simulink model "Six_phase_inverter"  (R2014b)
settings: Solver=ode23tb  StartTime=0.0  StopTime=0.05  MaxStep=1e-4  RelTol=1e-3
InitFcn:
  | Vm=100;
  | Fc=3000;
libraries: powerlib x12, simulink_extras x1, simulink x1
settings Model: Creator=y  LastModifiedBy=Lei
settings DataIOCC: SignalLoggingSaveFormat=ModelDataLogs
settings OptimizationCC: ExpressionDepthLimit=2147483647  InitFltsAndDblsToZero=on
settings DebuggingCC: SaveWithParameterizedLinksMsg=none  UnderspecifiedInitializationDetection=Classic  MergeDetectMultiDrivingBlocksExec=none  SignalResolutionControl=TryResolveAllWithWarning  MultiTaskDSMMsg=warning  MultiTaskCondExecSysMsg=none  FcnCallInpInsideContextMsg=UseLocalSettings  StateNameClashWarn=warning
settings RTWCC: IncludeERTFirstTime=on
settings GRTTargetCC: TargetFcnLib=ansi_tfl_tmw.mat  CombineOutputUpdateFcns=off  GRTInterface=on

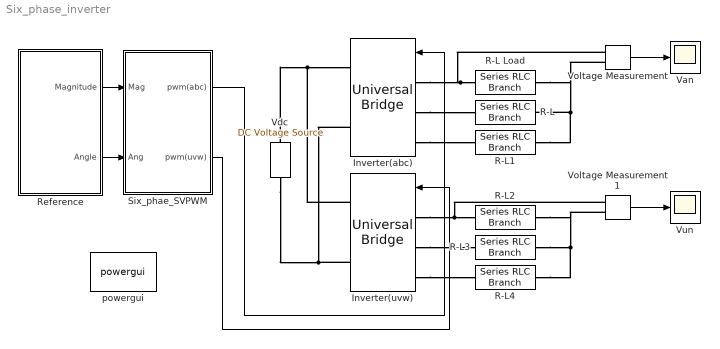
== system Six_phase_inverter ==
  Inverter(abc) : powerlib/Power Electronics/Universal Bridge  Arms=3  SnubberResistance=1e5  SnubberCapacitance=inf  Device=IGBT / Diodes  Ron=1e-3  Lon=0  ForwardVoltages="[  0  0  ]"  ForwardVoltage=0  GTOparameters=[ 10e-6 , 20e-6 ]  IGBTparameters=[ 1e-6 , 2e-6 ]  Measurements=None  Measurements_2=None  converterType=Rectifier
  Inverter(uvw) : powerlib/Power Electronics/Universal Bridge  Arms=3  SnubberResistance=1e5  SnubberCapacitance=inf  Device=IGBT / Diodes  Ron=1e-3  Lon=0  ForwardVoltages="[  0  0  ]"  ForwardVoltage=0  GTOparameters=[ 10e-6 , 20e-6 ]  IGBTparameters=[ 1e-6 , 2e-6 ]  Measurements=None  Measurements_2=None  converterType=Rectifier
  R-L{,1..4} (5 alike) : powerlib/Elements/Series RLC Branch  LConnTagsString=__new0  RConnTagsString=__new0  BranchType=RL  Resistance=10  Inductance=1e-03  SetiL0=off  InitialCurrent=0  Capacitance=[]  Setx0=off  InitialVoltage=0  Measurements=None
  R-L Load : powerlib/Elements/Series RLC Branch  LConnTagsString=__new0  RConnTagsString=__new0  BranchType=RL  Resistance=10  Inductance=1e-03  SetiL0=off  InitialCurrent=0  Capacitance=[]  Setx0=off  InitialVoltage=0  Measurements=None
  Reference : Subsystem
      mask Display:
      | disp('reference\nvoltage\ngenerator')
      | port_label('output',1,'mag')
      | port_label('output',2,'angle')
  Six_phae_SVPWM : Subsystem
  Van : Scope
      settings: TimeRange=0.05  YMin=-200  YMax=200  SaveName=Van  SampleInput=on  SampleTime=1e-6
  Vdc : powerlib/Electrical Sources/DC Voltage Source  Amplitude=300  Measurements=None
  Voltage Measurement : powerlib/Measurements/Voltage Measurement  PhasorSimulation=off  OutputType=Complex  PSBequivalent=0
  Voltage Measurement1 : powerlib/Measurements/Voltage Measurement  PhasorSimulation=off  OutputType=Complex  PSBequivalent=0
  Vun : Scope
      settings: YMin=-200  YMax=200  SaveName=Vbn  SampleInput=on  SampleTime=1e-6
  powergui : powerlib/powergui  Priority=1  SimulationMode=Continuous  SolverType=Tustin/Backward Euler (TBE)  SampleTime=50e-6  frequency=60  SPID=off  DisableSnubberDevices=off  DisableRonSwitches=off  DisableVfSwitches=off  SwTol=0  DisplayEquations=off  Interpol=off  methode=off  Ts=100  frequencyindice=0  Pbase=100e6  ErrMax=1e-4  Iterations=50  UnitsV=kV  UnitsW=MW  FunctionMessages=off  echomessages=off  HookPort=off  EnableUseOfTLC=off  x0status=blocks  RestoreLinks=warning  ResistiveCurrentMeasurement=off  Frange=[0:2:500]  Ylog=off  Xlog=on  ShowGrid=off  save=off  variable=ZData  structure=0  ZoomFFT=off  StartTime=0.0  cycles=1  DisplayStyle=1  fundamental=60  FreqAxis=off  MaxFrequency=1000  frequencyindicesteady=1  RmsSteady=1  display=off
  wires:
  Voltage Measurement/1 -> Van/1
  Reference/2(Angle) -> Six_phae_SVPWM/2(Ang)
  Reference/1(Magnitude) -> Six_phae_SVPWM/1(Mag)
  Voltage Measurement1/1 -> Vun/1
  Six_phae_SVPWM/1(pwm(abc)) -> Inverter(abc)/1
  Six_phae_SVPWM/2(pwm(uvw)) -> Inverter(uvw)/1
  connections:
  R-L Load/LConn1 -- Inverter(abc)/LConn1 -- Voltage Measurement/LConn1
  Inverter(abc)/LConn2 -- R-L/LConn1
  Inverter(abc)/LConn3 -- R-L1/LConn1
  Voltage Measurement1/LConn1 -- Inverter(uvw)/LConn1 -- R-L2/LConn1
  Inverter(uvw)/LConn2 -- R-L3/LConn1
  Inverter(uvw)/LConn3 -- R-L4/LConn1
  R-L4/RConn1 -- Voltage Measurement1/LConn2 -- R-L2/RConn1 -- R-L3/RConn1
  R-L1/RConn1 -- Voltage Measurement/LConn2 -- R-L Load/RConn1 -- R-L/RConn1
  Vdc/RConn1 -- Inverter(uvw)/RConn1 -- Inverter(abc)/RConn1
  Vdc/LConn1 -- Inverter(uvw)/RConn2 -- Inverter(abc)/RConn2

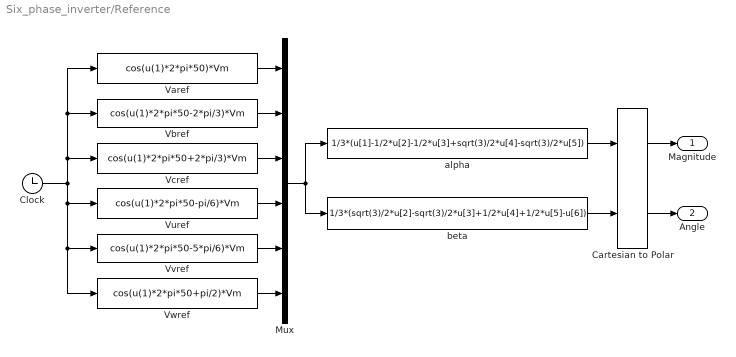
== system Six_phase_inverter/Reference ==
  Cartesian to Polar : simulink_extras/Transformations/Cartesian to Polar
  Clock : Clock
  Mux : Mux  Inputs=6
  Varef : Fcn  Expr=cos(u(1)*2*pi*50)*Vm
  Vbref : Fcn  Expr=cos(u(1)*2*pi*50-2*pi/3)*Vm
  Vcref : Fcn  Expr=cos(u(1)*2*pi*50+2*pi/3)*Vm
  Vuref : Fcn  Expr=cos(u(1)*2*pi*50-pi/6)*Vm
  Vvref : Fcn  Expr=cos(u(1)*2*pi*50-5*pi/6)*Vm
  Vwref : Fcn  Expr=cos(u(1)*2*pi*50+pi/2)*Vm
  alpha : Fcn  Expr=1/3*(u[1]-1/2*u[2]-1/2*u[3]+sqrt(3)/2*u[4]-sqrt(3)/2*u[5])
  beta : Fcn  Expr=1/3*(sqrt(3)/2*u[2]-sqrt(3)/2*u[3]+1/2*u[4]+1/2*u[5]-u[6])
  Magnitude : Outport
  Angle : Outport  Port=2
  wires:
  Varef/1 -> Mux/1
  Cartesian to Polar/1 -> Magnitude/1
  Cartesian to Polar/2 -> Angle/1
  Clock/1 -> Varef/1, Vbref/1, Vcref/1, Vwref/1, Vvref/1, Vuref/1
  Vbref/1 -> Mux/2
  Vcref/1 -> Mux/3
  Vvref/1 -> Mux/5
  Vwref/1 -> Mux/6
  Vuref/1 -> Mux/4
  Mux/1 -> alpha/1, beta/1
  beta/1 -> Cartesian to Polar/2
  alpha/1 -> Cartesian to Polar/1

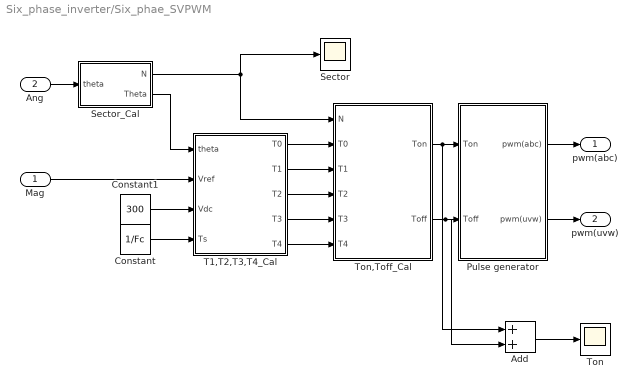
== system Six_phase_inverter/Six_phae_SVPWM ==
  Mag : Inport
  Ang : Inport  Port=2
  Add : Sum
  Constant : Constant  Value=1/Fc
  Constant1 : Constant  Value=300
  Pulse generator : Subsystem
  Sector : Scope
      settings: YMin=0  YMax=12  SaveName=N  SampleInput=on  SampleTime=1e-6
  Sector_Cal : Subsystem
  T1,T2,T3,T4_Cal : MATLAB Function  TreatAsAtomicUnit=on
  Ton : Scope
      settings: YMin=0  YMax=12  SaveName=Ton  SampleInput=on  SampleTime=1e-6
  Ton,Toff_Cal : MATLAB Function  TreatAsAtomicUnit=on
  pwm(abc) : Outport
  pwm(uvw) : Outport  Port=2
  wires:
  Sector_Cal/1(N) -> Ton,Toff_Cal/1(N), Sector/1
  Sector_Cal/2(Theta) -> T1,T2,T3,T4_Cal/1(theta)
  Constant1/1 -> T1,T2,T3,T4_Cal/3(Vdc)
  Constant/1 -> T1,T2,T3,T4_Cal/4(Ts)
  T1,T2,T3,T4_Cal/1(T0) -> Ton,Toff_Cal/2(T0)
  T1,T2,T3,T4_Cal/2(T1) -> Ton,Toff_Cal/3(T1)
  T1,T2,T3,T4_Cal/3(T2) -> Ton,Toff_Cal/4(T2)
  T1,T2,T3,T4_Cal/4(T3) -> Ton,Toff_Cal/5(T3)
  T1,T2,T3,T4_Cal/5(T4) -> Ton,Toff_Cal/6(T4)
  Ton,Toff_Cal/1(Ton) -> Add/1, Pulse generator/1(Ton)
  Ton,Toff_Cal/2(Toff) -> Add/2, Pulse generator/2(Toff)
  Ang/1 -> Sector_Cal/1(theta)
  Mag/1 -> T1,T2,T3,T4_Cal/2(Vref)
  Pulse generator/2(pwm(uvw)) -> pwm(uvw)/1
  Pulse generator/1(pwm(abc)) -> pwm(abc)/1
  Add/1 -> Ton/1

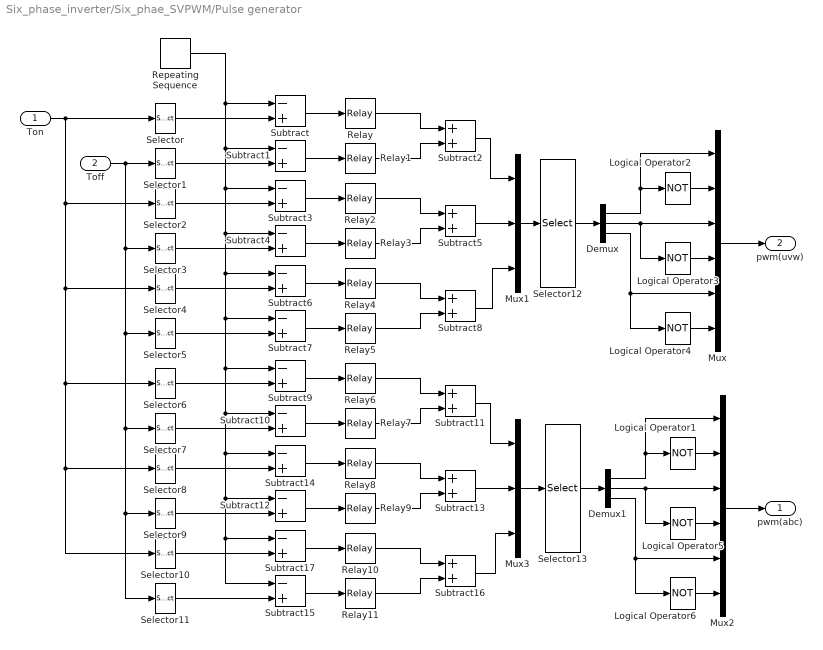
== system Six_phase_inverter/Six_phae_SVPWM/Pulse generator ==
  Ton : Inport
  Toff : Inport  Port=2
  Demux : Demux  Outputs=3
  Demux1 : Demux  Outputs=3
  Logical Operator{1..6} (6 alike) : Logic  Operator=NOT  OutDataTypeStr=float('double')
  Mux : Mux  Inputs=6
  Mux1 : Mux  Inputs=3
  Mux2 : Mux  Inputs=6
  Mux3 : Mux  Inputs=3
  Relay : Relay  OffSwitchValue=-eps
  Relay{1,3,5,7,9,11} (6 alike) : Relay  OnOutputValue=0  OffOutputValue=-1
  Relay{2,4,6,8,10} (5 alike) : Relay
  Repeating Sequence : simulink/Sources/Repeating Sequence  rep_seq_t=[0 0.5/Fc 1/Fc]  rep_seq_y=[0 0.5/Fc 0]
  Selector : Selector  InputPortWidth=6  Indices=[1]
  Selector1 : Selector  InputPortWidth=6  Indices=[1]
  Selector10 : Selector  InputPortWidth=6  Indices=[6]
  Selector11 : Selector  InputPortWidth=6  Indices=[6]
  Selector12 : Selector  InputPortWidth=3  Indices=[3 2 1]
  Selector13 : Selector  InputPortWidth=3  Indices=[3 2 1]
  Selector2 : Selector  InputPortWidth=6  Indices=[2]
  Selector3 : Selector  InputPortWidth=6  Indices=[2]
  Selector4 : Selector  InputPortWidth=6  Indices=[3]
  Selector5 : Selector  InputPortWidth=6  Indices=[3]
  Selector6 : Selector  InputPortWidth=6  Indices=[4]
  Selector7 : Selector  InputPortWidth=6  Indices=[4]
  Selector8 : Selector  InputPortWidth=6  Indices=[5]
  Selector9 : Selector  InputPortWidth=6  Indices=[5]
  Subtract{,1,3..4,6..7,9..10,12,14..15,17} (12 alike) : Sum  Inputs=-+
  Subtract{2,5,8,11,13,16} (6 alike) : Sum
  pwm(abc) : Outport
  pwm(uvw) : Outport  Port=2
  wires:
  Ton/1 -> Selector/1, Selector2/1, Selector4/1, Selector6/1, Selector8/1, Selector10/1
  Repeating Sequence/1 -> Subtract/1, Subtract1/1, Subtract3/1, Subtract4/1, Subtract6/1, Subtract7/1, Subtract9/1, Subtract10/1, Subtract14/1, Subtract12/1, Subtract15/1, Subtract17/1
  Subtract/1 -> Relay/1
  Toff/1 -> Selector9/1, Selector11/1, Selector7/1, Selector5/1, Selector3/1, Selector1/1
  Subtract1/1 -> Relay1/1
  Selector/1 -> Subtract/2
  Selector1/1 -> Subtract1/2
  Relay/1 -> Subtract2/1
  Relay1/1 -> Subtract2/2
  Subtract2/1 -> Mux1/1
  Subtract3/1 -> Relay2/1
  Subtract4/1 -> Relay3/1
  Selector2/1 -> Subtract3/2
  Selector3/1 -> Subtract4/2
  Relay2/1 -> Subtract5/1
  Relay3/1 -> Subtract5/2
  Subtract5/1 -> Mux1/2
  Subtract6/1 -> Relay4/1
  Subtract7/1 -> Relay5/1
  Selector4/1 -> Subtract6/2
  Selector5/1 -> Subtract7/2
  Relay4/1 -> Subtract8/1
  Relay5/1 -> Subtract8/2
  Subtract8/1 -> Mux1/3
  Subtract9/1 -> Relay6/1
  Subtract10/1 -> Relay7/1
  Selector6/1 -> Subtract9/2
  Selector7/1 -> Subtract10/2
  Relay6/1 -> Subtract11/1
  Relay7/1 -> Subtract11/2
  Subtract11/1 -> Mux3/1
  Subtract14/1 -> Relay8/1
  Subtract12/1 -> Relay9/1
  Selector8/1 -> Subtract14/2
  Selector9/1 -> Subtract12/2
  Relay8/1 -> Subtract13/1
  Relay9/1 -> Subtract13/2
  Subtract13/1 -> Mux3/2
  Subtract17/1 -> Relay10/1
  Subtract15/1 -> Relay11/1
  Selector10/1 -> Subtract17/2
  Selector11/1 -> Subtract15/2
  Relay10/1 -> Subtract16/1
  Relay11/1 -> Subtract16/2
  Subtract16/1 -> Mux3/3
  Logical Operator2/1 -> Mux/2
  Logical Operator3/1 -> Mux/4
  Logical Operator4/1 -> Mux/6
  Mux/1 -> pwm(uvw)/1
  Mux1/1 -> Selector12/1
  Selector12/1 -> Demux/1
  Demux/1 -> Mux/1, Logical Operator2/1
  Demux/2 -> Mux/3, Logical Operator3/1
  Demux/3 -> Mux/5, Logical Operator4/1
  Logical Operator1/1 -> Mux2/2
  Logical Operator5/1 -> Mux2/4
  Logical Operator6/1 -> Mux2/6
  Mux2/1 -> pwm(abc)/1
  Mux3/1 -> Selector13/1
  Selector13/1 -> Demux1/1
  Demux1/1 -> Mux2/1, Logical Operator1/1
  Demux1/2 -> Mux2/3, Logical Operator5/1
  Demux1/3 -> Mux2/5, Logical Operator6/1

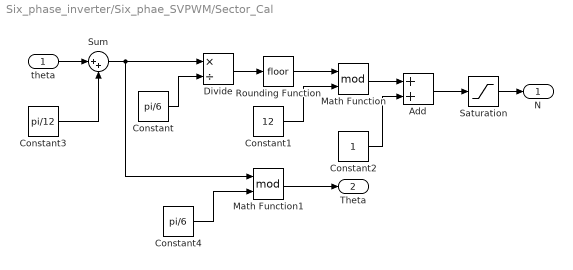
== system Six_phase_inverter/Six_phae_SVPWM/Sector_Cal ==
  theta : Inport
  Add : Sum
  Constant : Constant  Value=pi/6
  Constant1 : Constant  Value=12
  Constant2 : Constant
  Constant3 : Constant  Value=pi/12
  Constant4 : Constant  Value=pi/6
  Divide : Product  Inputs=*/
  Math Function : Math  Operator=mod  SaturateOnIntegerOverflow=on
  Math Function1 : Math  Operator=mod  SaturateOnIntegerOverflow=on
  Rounding Function : Rounding
  Saturation : Saturate  UpperLimit=12  LowerLimit=1
  Sum : Sum  Inputs=|++
  N : Outport
  Theta : Outport  Port=2
  wires:
  Constant/1 -> Divide/2
  Divide/1 -> Rounding Function/1
  Rounding Function/1 -> Math Function/1
  Constant1/1 -> Math Function/2
  Math Function/1 -> Add/1
  Constant2/1 -> Add/2
  Add/1 -> Saturation/1
  Saturation/1 -> N/1
  theta/1 -> Sum/1
  Sum/1 -> Math Function1/1, Divide/1
  Constant3/1 -> Sum/2
  Constant4/1 -> Math Function1/2
  Math Function1/1 -> Theta/1

== matlab function Six_phase_inverter/Six_phae_SVPWM/T1,T2,T3,T4_Cal ==
  data: theta input; Vref input; Vdc input; T0 output; Ts input; T1 output; T2 output; T3 output; T4 output
function [T0,T1,T2,T3,T4] = fcn(theta,Vref,Vdc,Ts)
%#codegen

k = sqrt(3)*(sqrt(3)-1)/(2*sqrt(2))/Vdc*Vref*Ts;
m = sin(pi/6-theta);
n = sin(theta);

A = k*m; %T1
B = k*(sqrt(3)*m+n);%T2
C = k*(m+sqrt(3)*n); %T3
D = k*n;            %T4

if A+B+C+D>Ts
    T1 = A/(A+B+C+D)*Ts;
    T2 = B/(A+B+C+D)*Ts;
    T3 = C/(A+B+C+D)*Ts;
    T4 = D/(A+B+C+D)*Ts;
    T0 = Ts-T1-T2-T3-T4;
else
    T1 = A;
    T2 = B;
    T3 = C;
    T4 = D;
    T0 = Ts-T1-T2-T3-T4;
end
end

== matlab function Six_phase_inverter/Six_phae_SVPWM/Ton,Toff_Cal ==
  data: N input; T0 input; T1 input; T2 input; T3 input; T4 input; Ton output; Toff output
function [Ton,Toff] = fcn(N,T0,T1,T2,T3,T4)
%#codegen
t01 = 1/4*T0;
t02 = 1/2*T0;

ta1 = t01;
tb1 = ta1+T2;
tc1 = tb1+T1;
td1 = tc1+t02;
te1 = td1+T4;
tf1 = te1+T3;

ta2 = t01;
tb2 = ta2+T1;
tc2 = tb2+T2;
td2 = tc2+t02;
te2 = td2+T3;
tf2 = te2+T4;

Ton = zeros(6,1);
Toff = zeros(6,1);

switch (N)
    case 1
        Ton(1) = ta1;Ton(2) = tc1; Ton(3) = ta1; 
        Ton(4) = tb1;Ton(5) = tc1; Ton(6) = ta1;
        Toff(1) = td1;Toff(2) = td1;Toff(3) = tf1;
        Toff(4) = td1;Toff(5) = te1;Toff(6) = tf1;
    case 2
        Ton(1) = tb1;Ton(2) = tc1; Ton(3) = ta1; 
        Ton(4) = tc1;Ton(5) = tc1; Ton(6) = ta1;
        Toff(1) = td1;Toff(2) = te1;Toff(3) = tf1;
        Toff(4) = td1;Toff(5) = tf1;Toff(6) = tf1;
   case 3
        Ton(1) = tc2;Ton(2) = tc2; Ton(3) = ta2; 
        Ton(4) = tc2;Ton(5) = tb2; Ton(6) = ta2;
        Toff(1) = td2;Toff(2) = tf2;Toff(3) = tf2;
        Toff(4) = td2;Toff(5) = tf2;Toff(6) = te2;
    case 4
        Ton(1) = tc2;Ton(2) = tb2; Ton(3) = ta2; 
        Ton(4) = tc2;Ton(5) = ta2; Ton(6) = ta2;
        Toff(1) = td2;Toff(2) = tf2;Toff(3) = te2;
        Toff(4) = td2;Toff(5) = tf2;Toff(6) = td2;
    case 5
        Ton(1) = tc1;Ton(2) = ta1; Ton(3) = ta1; 
        Ton(4) = tc1;Ton(5) = ta1; Ton(6) = tb1;
        Toff(1) = td1;Toff(2) = tf1;Toff(3) = td1;
        Toff(4) = te1;Toff(5) = tf1;Toff(6) = td1;
    case 6
        Ton(1) = tc1;Ton(2) = ta1; Ton(3) = tb1; 
        Ton(4) = tc1;Ton(5) = ta1; Ton(6) = tc1;
        Toff(1) = te1;Toff(2) = tf1;Toff(3) = td1;
        Toff(4) = tf1;Toff(5) = tf1;Toff(6) = td1;
    case 7
        Ton(1) = tc2;Ton(2) = ta2; Ton(3) = tc2; 
        Ton(4) = tb2;Ton(5) = ta2; Ton(6) = tc2;
        Toff(1) = tf2;Toff(2) = tf2;Toff(3) = td2;
        Toff(4) = tf2;Toff(5) = te2;Toff(6) = td2;
    case 8
        Ton(1) = tb2;Ton(2) = ta2; Ton(3) = tc2; 
        Ton(4) = ta2;Ton(5) = ta2; Ton(6) = tc2;
        Toff(1) = tf2;Toff(2) = te2;Toff(3) = td2;
        Toff(4) = tf2;Toff(5) = td2;Toff(6) = td2;
    case 9
        Ton(1) = ta1;Ton(2) = ta1; Ton(3) = tc1; 
        Ton(4) = ta1;Ton(5) = tb1; Ton(6) = tc1;
        Toff(1) = tf1;Toff(2) = td1;Toff(3) = td1;
        Toff(4) = tf1;Toff(5) = td1;Toff(6) = te1;
    case 10
        Ton(1) = ta1;Ton(2) = tb1; Ton(3) = tc1; 
        Ton(4) = ta1;Ton(5) = tc1; Ton(6) = tc1;
        Toff(1) = tf1;Toff(2) = td1;Toff(3) = te1;
        Toff(4) = tf1;Toff(5) = td1;Toff(6) = tf1;
    case 11
        Ton(1) = ta2;Ton(2) = tc2; Ton(3) = tc2; 
        Ton(4) = ta2;Ton(5) = tc2; Ton(6) = tb2;
        Toff(1) = tf2;Toff(2) = td2;Toff(3) = tf2;
        Toff(4) = te2;Toff(5) = td2;Toff(6) = tf2;
    case 12
        Ton(1) = ta2;Ton(2) = tc2; Ton(3) = tb2; 
        Ton(4) = ta2;Ton(5) = tc2; Ton(6) = ta2;
        Toff(1) = te2;Toff(2) = td2;Toff(3) = tf2;
        Toff(4) = td2;Toff(5) = td2;Toff(6) = tf2;       
end
end
